simulink model "Model_DesktopSim"  (R2016b)
settings: Solver=ode3  StartTime=0.0  StopTime=180  FixedStep=Ts  MaxStep=Ts  RelTol=1e-4  EnableMultiTasking=on
InitFcn:
  | initSimScript();
values from neighbouring files (symbols this model uses):
  Ts = 80e-6*2    (= 0.00016)    [initSimScript.m]
undefined symbols (not defined in the file or in its folder): DiscIntNeverNeededParam
libraries: cables_lib x34, modbus_lib x21, simulink x18, transformer_lib x13, dynamic_load_lib x12, powerlib x6, discretizing x4, Batt_lib x1, PV_lib x1
(part 1 of 3)
settings Model: SimulationMode=accelerator  Creator=jlesage  LastModifiedBy=jlesage
settings SolverCC: EnableConcurrentExecution=on
settings DataIOCC: SaveFormat=StructureWithTime
settings OptimizationCC: BlockReduction=off  OptimizeBlockIOStorage=off  BufferReuse=off  GlobalBufferReuse=off  ExpressionFolding=off  LocalBlockOutputs=off
settings DebuggingCC: ParameterPrecisionLossMsg=none
settings HardwareCC: ProdBitPerPointer=32  ProdBitPerSizeT=32  ProdBitPerPtrDiffT=32  ProdLargestAtomicFloat=None  ProdWordSize=32  ProdLongLongMode=on  ProdHWDeviceType=Generic->32-bit x86 compatible
settings RTWCC: SystemTargetFile=slrt.tlc  TemplateMakefile=slrt_default_tmf  Description=Simulink Real-Time  RTWCompilerOptimization=on

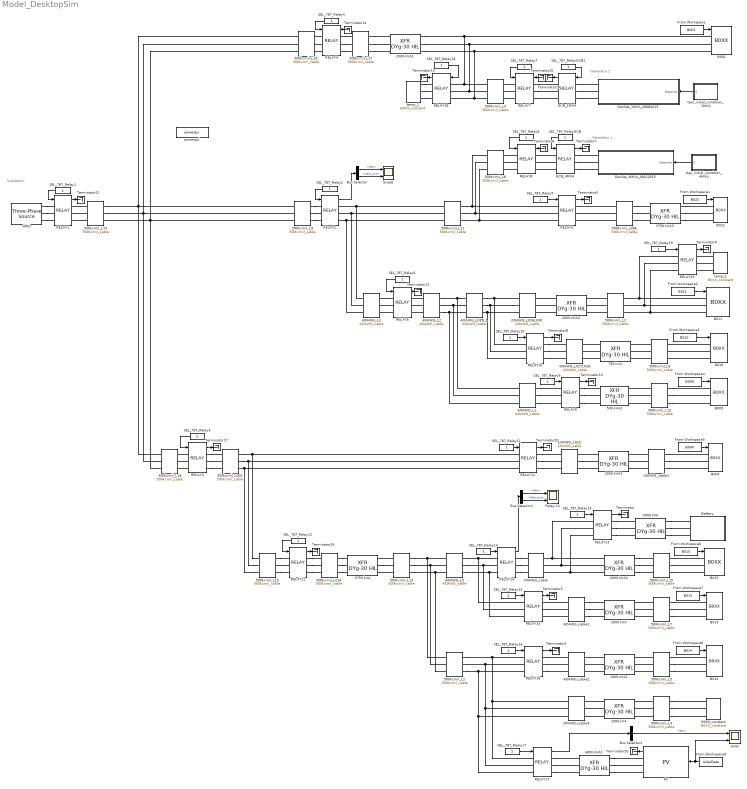
== system Model_DesktopSim ==
  note: Generator 2
  note: Generator 1
  note: Substation
  1/0AWG_L022 : cables_lib/1//0AWG_cable  length=1000  par_sets=1
  1/0AWG_cable1 : cables_lib/1//0AWG_cable  length=51  par_sets=1
  1000 kVA : transformer_lib/XFR DYg-30 HIL  Rating=1000  Vp=4160  Vs=460  Z=5.18  XR=2.5
  1000 kVA1 : transformer_lib/XFR DYg-30 HIL  Rating=1000  Vp=4160  Vs=216  Z=5.18  XR=2.5
  2/0AWG_L026L030 : cables_lib/2//0AWG_cable  length=1010  par_sets=1
  2000 kVA : transformer_lib/XFR DYg-30 HIL  Rating=2000  Vp=4160  Vs=216  Z=5.18  XR=2.5
  2000 kVA1 : transformer_lib/XFR DYg-30 HIL  Rating=2000  Vp=13800  Vs=460  Z=5.75  XR=5.7
  2000 kVA2 : transformer_lib/XFR DYg-30 HIL  Rating=2000  Vp=13800  Vs=460  Z=5.75  XR=5.7
  2000 kVA3 : transformer_lib/XFR DYg-30 HIL  Rating=2000  Vp=13800  Vs=460  Z=5.18  XR=2.5
  2000 kVA4 : transformer_lib/XFR DYg-30 HIL  Rating=2000  Vp=4160  Vs=216  Z=5.18  XR=2.5
  3750 kVA : transformer_lib/XFR DYg-30 HIL  Rating=3750  Vp=13800  Vs=4160  Z=4.75  XR=11.4
  3750 kVA3 : transformer_lib/XFR DYg-30 HIL  Rating=3750  Vp=13800  Vs=460  Z=4.75  XR=11.4
  4/0AWG_L027L028 : cables_lib/4//0AWG_cable  length=100  par_sets=1
  4/0AWG_L035L1 : cables_lib/4//0AWG_cable  length=1400  par_sets=1
  4/0AWG_L1 : cables_lib/4//0AWG_cable  length=25  par_sets=1
  4/0AWG_L2 : cables_lib/4//0AWG_cable  length=10  par_sets=1
  4/0AWG_L3 : cables_lib/4//0AWG_cable  length=150  par_sets=1
  4/0AWG_L5 : cables_lib/4//0AWG_cable  length=20  par_sets=1
  4/0AWG_cable{,1..3} (4 alike) : cables_lib/4//0AWG_cable  length=51  par_sets=1
  4000 kVA : transformer_lib/XFR DYg-30 HIL  Rating=4000  Vp=2047  Vs=4160  Z=6.37  XR=3.5
  4000 kVA1 : transformer_lib/XFR DYg-30 HIL  Rating=4000  Vp=2047  Vs=4160  Z=6.37  XR=3.5
  500 kVA2 : transformer_lib/XFR DYg-30 HIL  Rating=500  Vp=13800  Vs=460  Z=5  XR=4.9
  500kcmil_L002 : cables_lib/500kcmil_cable  length=1851  par_sets=1
  500kcmil_L006 : cables_lib/500kcmil_cable  length=251  par_sets=1
  500kcmil_L018 : cables_lib/500kcmil_cable  length=1851  par_sets=1
  500kcmil_L{1,6,15..16} (4 alike) : cables_lib/500kcmil_cable  length=50  par_sets=1
  500kcmil_L{4..5,7,10} (4 alike) : cables_lib/500kcmil_cable  length=25  par_sets=1
  500kcmil_L11 : cables_lib/500kcmil_cable  length=21  par_sets=1
  500kcmil_L12 : cables_lib/500kcmil_cable  length=50  par_sets=2
  500kcmil_L13 : cables_lib/500kcmil_cable  length=51  par_sets=1
  500kcmil_L14 : cables_lib/500kcmil_cable  length=350  par_sets=1
  500kcmil_L17 : cables_lib/500kcmil_cable  length=1000  par_sets=1
  500kcmil_L18 : cables_lib/500kcmil_cable  length=51  par_sets=1
  500kcmil_L2 : cables_lib/500kcmil_cable  length=125  par_sets=2
  500kcmil_L3 : cables_lib/500kcmil_cable  length=60  par_sets=1
  500kcmil_L8 : cables_lib/500kcmil_cable  length=100  par_sets=1
  500kcmil_L9 : cables_lib/500kcmil_cable  length=720  par_sets=1
  750 kVA : transformer_lib/XFR DYg-30 HIL  Rating=750  Vp=13800  Vs=460  Z=5.57  XR=3.96
  B001 : dynamic_load_lib/B0XX  V=460  P_Scale=2  Q_Scale=2
  B003_constant : dynamic_load_lib/B0XX_constant  v=460  kVA=60  pf=0.9
  B004 : dynamic_load_lib/B0XX  V=460  P_Scale=2  Q_Scale=2
  B009 : dynamic_load_lib/B0XX  V=460  P_Scale=2  Q_Scale=2
  B010 : dynamic_load_lib/B0XX  V=460  P_Scale=1  Q_Scale=1
  B011 : dynamic_load_lib/B0XX  V=460  P_Scale=1  Q_Scale=1
  B013 : dynamic_load_lib/B0XX  V=208  P_Scale=2  Q_Scale=2
  B014 : dynamic_load_lib/B0XX  V=208  P_Scale=1  Q_Scale=1
  B015 : dynamic_load_lib/B0XX  V=208  P_Scale=2  Q_Scale=2
  B022 : dynamic_load_lib/B0XX  V=460  P_Scale=1  Q_Scale=1
  Battery : Subsystem
  Bus Selector : BusSelector  OutputSignals=Iabc,Vabc_bus
  Bus Selector1 : BusSelector  OutputSignals=Iabc,Vabc_bus
  Bus Selector2 : BusSelector  OutputSignals=Iabc
  From Workspace : FromWorkspace  VariableName=B001  SampleTime=Ts  OutputAfterFinalValue=Holding final value
  From Workspace1 : FromWorkspace  VariableName=B022  SampleTime=Ts  OutputAfterFinalValue=Holding final value
  From Workspace2 : FromWorkspace  VariableName=B011  SampleTime=Ts  OutputAfterFinalValue=Holding final value
  From Workspace3 : FromWorkspace  VariableName=B010  SampleTime=Ts  OutputAfterFinalValue=Holding final value
  From Workspace4 : FromWorkspace  VariableName=B009  SampleTime=Ts  OutputAfterFinalValue=Holding final value
  From Workspace5 : FromWorkspace  VariableName=B004  SampleTime=Ts  OutputAfterFinalValue=Holding final value
  From Workspace6 : FromWorkspace  VariableName=B015  SampleTime=Ts  OutputAfterFinalValue=Holding final value
  From Workspace7 : FromWorkspace  VariableName=B013  SampleTime=Ts  OutputAfterFinalValue=Holding final value
  From Workspace8 : FromWorkspace  VariableName=B014  SampleTime=Ts  OutputAfterFinalValue=Holding final value
  From Workspace9 : FromWorkspace  VariableName=solarData  SampleTime=Ts  OutputAfterFinalValue=Holding final value
  GCB_1MVA : modbus_lib/RELAY  Ts=Ts
      link override Three-Phase V-I Measurement/Model/VI/Ia: GotoTag=LibraryTag_Ia
      link override Three-Phase V-I Measurement/Model/VI/Ib: GotoTag=LibraryTag_Ib
      link override Three-Phase V-I Measurement/Model/VI/Ic: GotoTag=LibraryTag_Ic
      link override Three-Phase V-I Measurement/Model/VI/Va: GotoTag=LibraryTag_Va
      link override Three-Phase V-I Measurement/Model/VI/Vb: GotoTag=LibraryTag_Vb
      link override Three-Phase V-I Measurement/Model/VI/Vc: GotoTag=LibraryTag_Vc
      link override Three-Phase V-I Measurement1/Model/VI/Ia: GotoTag=LibraryTag_Ia
      link override Three-Phase V-I Measurement1/Model/VI/Ib: GotoTag=LibraryTag_Ib
      link override Three-Phase V-I Measurement1/Model/VI/Ic: GotoTag=LibraryTag_Ic
      link override Three-Phase V-I Measurement1/Model/VI/Va: GotoTag=LibraryTag_Va
      link override Three-Phase V-I Measurement1/Model/VI/Vb: GotoTag=LibraryTag_Vb
      link override Three-Phase V-I Measurement1/Model/VI/Vc: GotoTag=LibraryTag_Vc
  GCB_4MVA : modbus_lib/RELAY  Ts=Ts
      link override Three-Phase V-I Measurement/Model/VI/Ia: GotoTag=LibraryTag_Ia
      link override Three-Phase V-I Measurement/Model/VI/Ib: GotoTag=LibraryTag_Ib
      link override Three-Phase V-I Measurement/Model/VI/Ic: GotoTag=LibraryTag_Ic
      link override Three-Phase V-I Measurement/Model/VI/Va: GotoTag=LibraryTag_Va
      link override Three-Phase V-I Measurement/Model/VI/Vb: GotoTag=LibraryTag_Vb
      link override Three-Phase V-I Measurement/Model/VI/Vc: GotoTag=LibraryTag_Vc
      link override Three-Phase V-I Measurement1/Model/VI/Ia: GotoTag=LibraryTag_Ia
      link override Three-Phase V-I Measurement1/Model/VI/Ib: GotoTag=LibraryTag_Ib
      link override Three-Phase V-I Measurement1/Model/VI/Ic: GotoTag=LibraryTag_Ic
      link override Three-Phase V-I Measurement1/Model/VI/Va: GotoTag=LibraryTag_Va
      link override Three-Phase V-I Measurement1/Model/VI/Vb: GotoTag=LibraryTag_Vb
      link override Three-Phase V-I Measurement1/Model/VI/Vc: GotoTag=LibraryTag_Vc
  GRID : powerlib/Electrical Sources/Three-Phase Source  InternalConnection=Yg  VoltagePhases=off  Voltage=13970  PhaseAngle=0  Voltage_phases=[25e3 25e3 25e3]/sqrt(3)  PhaseAngles_phases=[0 -120 +120]  Frequency=60  NonIdealSource=on  SpecifyImpedance=on  Resistance=0.8929  Inductance=16.58e-3  ShortCircuitLevel=375e6  BaseVoltage=13800  XRratio=7.9  BusType=swing  Pref=0  Qref=0  Prefabc=[10e3, 10e3, 10e3]  Qrefabc=[0, 0, 0]  Qmin=-inf  Qmax=inf
  GenSet_1MVA_09082015 : Subsystem
  GenSet_4MVA_09212015 : Subsystem
  Gen_initial_condition_1MVA : Subsystem
  Gen_initial_condition_4MVA : Subsystem
  PV : PV_lib/PV  max_power=4e6  VacRMS=1200  VacRMS_limit_pu=[1.15 0.85]
  RELAY1 : modbus_lib/RELAY  Ts=Ts
      link override Three-Phase V-I Measurement/Model/VI/Ia: GotoTag=LibraryTag_Ia
      link override Three-Phase V-I Measurement/Model/VI/Ib: GotoTag=LibraryTag_Ib
      link override Three-Phase V-I Measurement/Model/VI/Ic: GotoTag=LibraryTag_Ic
      link override Three-Phase V-I Measurement/Model/VI/Va: GotoTag=LibraryTag_Va
      link override Three-Phase V-I Measurement/Model/VI/Vb: GotoTag=LibraryTag_Vb
      link override Three-Phase V-I Measurement/Model/VI/Vc: GotoTag=LibraryTag_Vc
      link override Three-Phase V-I Measurement1/Model/VI/Ia: GotoTag=LibraryTag_Ia
      link override Three-Phase V-I Measurement1/Model/VI/Ib: GotoTag=LibraryTag_Ib
      link override Three-Phase V-I Measurement1/Model/VI/Ic: GotoTag=LibraryTag_Ic
      link override Three-Phase V-I Measurement1/Model/VI/Va: GotoTag=LibraryTag_Va
      link override Three-Phase V-I Measurement1/Model/VI/Vb: GotoTag=LibraryTag_Vb
      link override Three-Phase V-I Measurement1/Model/VI/Vc: GotoTag=LibraryTag_Vc
  RELAY10 : modbus_lib/RELAY  Ts=Ts
      link override Three-Phase V-I Measurement/Model/VI/Ia: GotoTag=LibraryTag_Ia
      link override Three-Phase V-I Measurement/Model/VI/Ib: GotoTag=LibraryTag_Ib
      link override Three-Phase V-I Measurement/Model/VI/Ic: GotoTag=LibraryTag_Ic
      link override Three-Phase V-I Measurement/Model/VI/Va: GotoTag=LibraryTag_Va
      link override Three-Phase V-I Measurement/Model/VI/Vb: GotoTag=LibraryTag_Vb
      link override Three-Phase V-I Measurement/Model/VI/Vc: GotoTag=LibraryTag_Vc
      link override Three-Phase V-I Measurement1/Model/VI/Ia: GotoTag=LibraryTag_Ia
      link override Three-Phase V-I Measurement1/Model/VI/Ib: GotoTag=LibraryTag_Ib
      link override Three-Phase V-I Measurement1/Model/VI/Ic: GotoTag=LibraryTag_Ic
      link override Three-Phase V-I Measurement1/Model/VI/Va: GotoTag=LibraryTag_Va
      link override Three-Phase V-I Measurement1/Model/VI/Vb: GotoTag=LibraryTag_Vb
      link override Three-Phase V-I Measurement1/Model/VI/Vc: GotoTag=LibraryTag_Vc
  RELAY11 : modbus_lib/RELAY  Ts=Ts
      link override Three-Phase V-I Measurement/Model/VI/Ia: GotoTag=LibraryTag_Ia
      link override Three-Phase V-I Measurement/Model/VI/Ib: GotoTag=LibraryTag_Ib
      link override Three-Phase V-I Measurement/Model/VI/Ic: GotoTag=LibraryTag_Ic
      link override Three-Phase V-I Measurement/Model/VI/Va: GotoTag=LibraryTag_Va
      link override Three-Phase V-I Measurement/Model/VI/Vb: GotoTag=LibraryTag_Vb
      link override Three-Phase V-I Measurement/Model/VI/Vc: GotoTag=LibraryTag_Vc
      link override Three-Phase V-I Measurement1/Model/VI/Ia: GotoTag=LibraryTag_Ia
      link override Three-Phase V-I Measurement1/Model/VI/Ib: GotoTag=LibraryTag_Ib
      link override Three-Phase V-I Measurement1/Model/VI/Ic: GotoTag=LibraryTag_Ic
      link override Three-Phase V-I Measurement1/Model/VI/Va: GotoTag=LibraryTag_Va
      link override Three-Phase V-I Measurement1/Model/VI/Vb: GotoTag=LibraryTag_Vb
      link override Three-Phase V-I Measurement1/Model/VI/Vc: GotoTag=LibraryTag_Vc
  RELAY12 : modbus_lib/RELAY  Ts=Ts
      link override Three-Phase V-I Measurement/Model/VI/Ia: GotoTag=LibraryTag_Ia
      link override Three-Phase V-I Measurement/Model/VI/Ib: GotoTag=LibraryTag_Ib
      link override Three-Phase V-I Measurement/Model/VI/Ic: GotoTag=LibraryTag_Ic
      link override Three-Phase V-I Measurement/Model/VI/Va: GotoTag=LibraryTag_Va
      link override Three-Phase V-I Measurement/Model/VI/Vb: GotoTag=LibraryTag_Vb
      link override Three-Phase V-I Measurement/Model/VI/Vc: GotoTag=LibraryTag_Vc
      link override Three-Phase V-I Measurement1/Model/VI/Ia: GotoTag=LibraryTag_Ia
      link override Three-Phase V-I Measurement1/Model/VI/Ib: GotoTag=LibraryTag_Ib
      link override Three-Phase V-I Measurement1/Model/VI/Ic: GotoTag=LibraryTag_Ic
      link override Three-Phase V-I Measurement1/Model/VI/Va: GotoTag=LibraryTag_Va
      link override Three-Phase V-I Measurement1/Model/VI/Vb: GotoTag=LibraryTag_Vb
      link override Three-Phase V-I Measurement1/Model/VI/Vc: GotoTag=LibraryTag_Vc
  RELAY13 : modbus_lib/RELAY  Ts=Ts
  RELAY14 : modbus_lib/RELAY  Ts=Ts
      link override Three-Phase V-I Measurement/Model/VI/Ia: GotoTag=LibraryTag_Ia
      link override Three-Phase V-I Measurement/Model/VI/Ib: GotoTag=LibraryTag_Ib
      link override Three-Phase V-I Measurement/Model/VI/Ic: GotoTag=LibraryTag_Ic
      link override Three-Phase V-I Measurement/Model/VI/Va: GotoTag=LibraryTag_Va
      link override Three-Phase V-I Measurement/Model/VI/Vb: GotoTag=LibraryTag_Vb
      link override Three-Phase V-I Measurement/Model/VI/Vc: GotoTag=LibraryTag_Vc
      link override Three-Phase V-I Measurement1/Model/VI/Ia: GotoTag=LibraryTag_Ia
      link override Three-Phase V-I Measurement1/Model/VI/Ib: GotoTag=LibraryTag_Ib
      link override Three-Phase V-I Measurement1/Model/VI/Ic: GotoTag=LibraryTag_Ic
      link override Three-Phase V-I Measurement1/Model/VI/Va: GotoTag=LibraryTag_Va
      link override Three-Phase V-I Measurement1/Model/VI/Vb: GotoTag=LibraryTag_Vb
      link override Three-Phase V-I Measurement1/Model/VI/Vc: GotoTag=LibraryTag_Vc
  RELAY15 : modbus_lib/RELAY  Ts=Ts
      link override Three-Phase V-I Measurement/Model/VI/Ia: GotoTag=LibraryTag_Ia
      link override Three-Phase V-I Measurement/Model/VI/Ib: GotoTag=LibraryTag_Ib
      link override Three-Phase V-I Measurement/Model/VI/Ic: GotoTag=LibraryTag_Ic
      link override Three-Phase V-I Measurement/Model/VI/Va: GotoTag=LibraryTag_Va
      link override Three-Phase V-I Measurement/Model/VI/Vb: GotoTag=LibraryTag_Vb
      link override Three-Phase V-I Measurement/Model/VI/Vc: GotoTag=LibraryTag_Vc
      link override Three-Phase V-I Measurement1/Model/VI/Ia: GotoTag=LibraryTag_Ia
      link override Three-Phase V-I Measurement1/Model/VI/Ib: GotoTag=LibraryTag_Ib
      link override Three-Phase V-I Measurement1/Model/VI/Ic: GotoTag=LibraryTag_Ic
      link override Three-Phase V-I Measurement1/Model/VI/Va: GotoTag=LibraryTag_Va
      link override Three-Phase V-I Measurement1/Model/VI/Vb: GotoTag=LibraryTag_Vb
      link override Three-Phase V-I Measurement1/Model/VI/Vc: GotoTag=LibraryTag_Vc
  RELAY16 : modbus_lib/RELAY  Ts=Ts
      link override Three-Phase V-I Measurement/Model/VI/Ia: GotoTag=LibraryTag_Ia
      link override Three-Phase V-I Measurement/Model/VI/Ib: GotoTag=LibraryTag_Ib
      link override Three-Phase V-I Measurement/Model/VI/Ic: GotoTag=LibraryTag_Ic
      link override Three-Phase V-I Measurement/Model/VI/Va: GotoTag=LibraryTag_Va
      link override Three-Phase V-I Measurement/Model/VI/Vb: GotoTag=LibraryTag_Vb
      link override Three-Phase V-I Measurement/Model/VI/Vc: GotoTag=LibraryTag_Vc
      link override Three-Phase V-I Measurement1/Model/VI/Ia: GotoTag=LibraryTag_Ia
      link override Three-Phase V-I Measurement1/Model/VI/Ib: GotoTag=LibraryTag_Ib
      link override Three-Phase V-I Measurement1/Model/VI/Ic: GotoTag=LibraryTag_Ic
      link override Three-Phase V-I Measurement1/Model/VI/Va: GotoTag=LibraryTag_Va
      link override Three-Phase V-I Measurement1/Model/VI/Vb: GotoTag=LibraryTag_Vb
      link override Three-Phase V-I Measurement1/Model/VI/Vc: GotoTag=LibraryTag_Vc
  RELAY17 : modbus_lib/RELAY  Ts=Ts
      link override Three-Phase V-I Measurement/Model/VI/Ia: GotoTag=LibraryTag_Ia
      link override Three-Phase V-I Measurement/Model/VI/Ib: GotoTag=LibraryTag_Ib
      link override Three-Phase V-I Measurement/Model/VI/Ic: GotoTag=LibraryTag_Ic
      link override Three-Phase V-I Measurement/Model/VI/Va: GotoTag=LibraryTag_Va
      link override Three-Phase V-I Measurement/Model/VI/Vb: GotoTag=LibraryTag_Vb
      link override Three-Phase V-I Measurement/Model/VI/Vc: GotoTag=LibraryTag_Vc
      link override Three-Phase V-I Measurement1/Model/VI/Ia: GotoTag=LibraryTag_Ia
      link override Three-Phase V-I Measurement1/Model/VI/Ib: GotoTag=LibraryTag_Ib
      link override Three-Phase V-I Measurement1/Model/VI/Ic: GotoTag=LibraryTag_Ic
      link override Three-Phase V-I Measurement1/Model/VI/Va: GotoTag=LibraryTag_Va
      link override Three-Phase V-I Measurement1/Model/VI/Vb: GotoTag=LibraryTag_Vb
      link override Three-Phase V-I Measurement1/Model/VI/Vc: GotoTag=LibraryTag_Vc
  RELAY18 : modbus_lib/RELAY  Ts=Ts
      link override Three-Phase V-I Measurement/Model/VI/Ia: GotoTag=LibraryTag_Ia
      link override Three-Phase V-I Measurement/Model/VI/Ib: GotoTag=LibraryTag_Ib
      link override Three-Phase V-I Measurement/Model/VI/Ic: GotoTag=LibraryTag_Ic
      link override Three-Phase V-I Measurement/Model/VI/Va: GotoTag=LibraryTag_Va
      link override Three-Phase V-I Measurement/Model/VI/Vb: GotoTag=LibraryTag_Vb
      link override Three-Phase V-I Measurement/Model/VI/Vc: GotoTag=LibraryTag_Vc
      link override Three-Phase V-I Measurement1/Model/VI/Ia: GotoTag=LibraryTag_Ia
      link override Three-Phase V-I Measurement1/Model/VI/Ib: GotoTag=LibraryTag_Ib
      link override Three-Phase V-I Measurement1/Model/VI/Ic: GotoTag=LibraryTag_Ic
      link override Three-Phase V-I Measurement1/Model/VI/Va: GotoTag=LibraryTag_Va
      link override Three-Phase V-I Measurement1/Model/VI/Vb: GotoTag=LibraryTag_Vb
      link override Three-Phase V-I Measurement1/Model/VI/Vc: GotoTag=LibraryTag_Vc
  RELAY19 : modbus_lib/RELAY  Ts=Ts
      link override Three-Phase V-I Measurement/Model/VI/Ia: GotoTag=LibraryTag_Ia
      link override Three-Phase V-I Measurement/Model/VI/Ib: GotoTag=LibraryTag_Ib
      link override Three-Phase V-I Measurement/Model/VI/Ic: GotoTag=LibraryTag_Ic
      link override Three-Phase V-I Measurement/Model/VI/Va: GotoTag=LibraryTag_Va
      link override Three-Phase V-I Measurement/Model/VI/Vb: GotoTag=LibraryTag_Vb
      link override Three-Phase V-I Measurement/Model/VI/Vc: GotoTag=LibraryTag_Vc
      link override Three-Phase V-I Measurement1/Model/VI/Ia: GotoTag=LibraryTag_Ia
      link override Three-Phase V-I Measurement1/Model/VI/Ib: GotoTag=LibraryTag_Ib
      link override Three-Phase V-I Measurement1/Model/VI/Ic: GotoTag=LibraryTag_Ic
      link override Three-Phase V-I Measurement1/Model/VI/Va: GotoTag=LibraryTag_Va
      link override Three-Phase V-I Measurement1/Model/VI/Vb: GotoTag=LibraryTag_Vb
      link override Three-Phase V-I Measurement1/Model/VI/Vc: GotoTag=LibraryTag_Vc
  RELAY2 : modbus_lib/RELAY  Ts=Ts
      link override Three-Phase V-I Measurement/Model/VI/Ia: GotoTag=LibraryTag_Ia
      link override Three-Phase V-I Measurement/Model/VI/Ib: GotoTag=LibraryTag_Ib
      link override Three-Phase V-I Measurement/Model/VI/Ic: GotoTag=LibraryTag_Ic
      link override Three-Phase V-I Measurement/Model/VI/Va: GotoTag=LibraryTag_Va
      link override Three-Phase V-I Measurement/Model/VI/Vb: GotoTag=LibraryTag_Vb
      link override Three-Phase V-I Measurement/Model/VI/Vc: GotoTag=LibraryTag_Vc
      link override Three-Phase V-I Measurement1/Model/VI/Ia: GotoTag=LibraryTag_Ia
      link override Three-Phase V-I Measurement1/Model/VI/Ib: GotoTag=LibraryTag_Ib
      link override Three-Phase V-I Measurement1/Model/VI/Ic: GotoTag=LibraryTag_Ic
      link override Three-Phase V-I Measurement1/Model/VI/Va: GotoTag=LibraryTag_Va
      link override Three-Phase V-I Measurement1/Model/VI/Vb: GotoTag=LibraryTag_Vb
      link override Three-Phase V-I Measurement1/Model/VI/Vc: GotoTag=LibraryTag_Vc
  RELAY3 : modbus_lib/RELAY  Ts=Ts
      link override Three-Phase V-I Measurement/Model/VI/Ia: GotoTag=LibraryTag_Ia
      link override Three-Phase V-I Measurement/Model/VI/Ib: GotoTag=LibraryTag_Ib
      link override Three-Phase V-I Measurement/Model/VI/Ic: GotoTag=LibraryTag_Ic
      link override Three-Phase V-I Measurement/Model/VI/Va: GotoTag=LibraryTag_Va
      link override Three-Phase V-I Measurement/Model/VI/Vb: GotoTag=LibraryTag_Vb
      link override Three-Phase V-I Measurement/Model/VI/Vc: GotoTag=LibraryTag_Vc
      link override Three-Phase V-I Measurement1/Model/VI/Ia: GotoTag=LibraryTag_Ia
      link override Three-Phase V-I Measurement1/Model/VI/Ib: GotoTag=LibraryTag_Ib
      link override Three-Phase V-I Measurement1/Model/VI/Ic: GotoTag=LibraryTag_Ic
      link override Three-Phase V-I Measurement1/Model/VI/Va: GotoTag=LibraryTag_Va
      link override Three-Phase V-I Measurement1/Model/VI/Vb: GotoTag=LibraryTag_Vb
      link override Three-Phase V-I Measurement1/Model/VI/Vc: GotoTag=LibraryTag_Vc
  RELAY4 : modbus_lib/RELAY  Ts=Ts
      link override Three-Phase V-I Measurement/Model/VI/Ia: GotoTag=LibraryTag_Ia
      link override Three-Phase V-I Measurement/Model/VI/Ib: GotoTag=LibraryTag_Ib
      link override Three-Phase V-I Measurement/Model/VI/Ic: GotoTag=LibraryTag_Ic
      link override Three-Phase V-I Measurement/Model/VI/Va: GotoTag=LibraryTag_Va
      link override Three-Phase V-I Measurement/Model/VI/Vb: GotoTag=LibraryTag_Vb
      link override Three-Phase V-I Measurement/Model/VI/Vc: GotoTag=LibraryTag_Vc
      link override Three-Phase V-I Measurement1/Model/VI/Ia: GotoTag=LibraryTag_Ia
      link override Three-Phase V-I Measurement1/Model/VI/Ib: GotoTag=LibraryTag_Ib
      link override Three-Phase V-I Measurement1/Model/VI/Ic: GotoTag=LibraryTag_Ic
      link override Three-Phase V-I Measurement1/Model/VI/Va: GotoTag=LibraryTag_Va
      link override Three-Phase V-I Measurement1/Model/VI/Vb: GotoTag=LibraryTag_Vb
      link override Three-Phase V-I Measurement1/Model/VI/Vc: GotoTag=LibraryTag_Vc
  RELAY5 : modbus_lib/RELAY  Ts=Ts
      link override Three-Phase V-I Measurement/Model/VI/Ia: GotoTag=LibraryTag_Ia
      link override Three-Phase V-I Measurement/Model/VI/Ib: GotoTag=LibraryTag_Ib
      link override Three-Phase V-I Measurement/Model/VI/Ic: GotoTag=LibraryTag_Ic
      link override Three-Phase V-I Measurement/Model/VI/Va: GotoTag=LibraryTag_Va
      link override Three-Phase V-I Measurement/Model/VI/Vb: GotoTag=LibraryTag_Vb
      link override Three-Phase V-I Measurement/Model/VI/Vc: GotoTag=LibraryTag_Vc
      link override Three-Phase V-I Measurement1/Model/VI/Ia: GotoTag=LibraryTag_Ia
      link override Three-Phase V-I Measurement1/Model/VI/Ib: GotoTag=LibraryTag_Ib
      link override Three-Phase V-I Measurement1/Model/VI/Ic: GotoTag=LibraryTag_Ic
      link override Three-Phase V-I Measurement1/Model/VI/Va: GotoTag=LibraryTag_Va
      link override Three-Phase V-I Measurement1/Model/VI/Vb: GotoTag=LibraryTag_Vb
      link override Three-Phase V-I Measurement1/Model/VI/Vc: GotoTag=LibraryTag_Vc
  RELAY6 : modbus_lib/RELAY  Ts=Ts
      link override Three-Phase V-I Measurement/Model/VI/Ia: GotoTag=LibraryTag_Ia
      link override Three-Phase V-I Measurement/Model/VI/Ib: GotoTag=LibraryTag_Ib
      link override Three-Phase V-I Measurement/Model/VI/Ic: GotoTag=LibraryTag_Ic
      link override Three-Phase V-I Measurement/Model/VI/Va: GotoTag=LibraryTag_Va
      link override Three-Phase V-I Measurement/Model/VI/Vb: GotoTag=LibraryTag_Vb
      link override Three-Phase V-I Measurement/Model/VI/Vc: GotoTag=LibraryTag_Vc
      link override Three-Phase V-I Measurement1/Model/VI/Ia: GotoTag=LibraryTag_Ia
      link override Three-Phase V-I Measurement1/Model/VI/Ib: GotoTag=LibraryTag_Ib
      link override Three-Phase V-I Measurement1/Model/VI/Ic: GotoTag=LibraryTag_Ic
      link override Three-Phase V-I Measurement1/Model/VI/Va: GotoTag=LibraryTag_Va
      link override Three-Phase V-I Measurement1/Model/VI/Vb: GotoTag=LibraryTag_Vb
      link override Three-Phase V-I Measurement1/Model/VI/Vc: GotoTag=LibraryTag_Vc
  RELAY7 : modbus_lib/RELAY  Ts=Ts
      link override Three-Phase V-I Measurement/Model/VI/Ia: GotoTag=LibraryTag_Ia
      link override Three-Phase V-I Measurement/Model/VI/Ib: GotoTag=LibraryTag_Ib
      link override Three-Phase V-I Measurement/Model/VI/Ic: GotoTag=LibraryTag_Ic
      link override Three-Phase V-I Measurement/Model/VI/Va: GotoTag=LibraryTag_Va
      link override Three-Phase V-I Measurement/Model/VI/Vb: GotoTag=LibraryTag_Vb
      link override Three-Phase V-I Measurement/Model/VI/Vc: GotoTag=LibraryTag_Vc
      link override Three-Phase V-I Measurement1/Model/VI/Ia: GotoTag=LibraryTag_Ia
      link override Three-Phase V-I Measurement1/Model/VI/Ib: GotoTag=LibraryTag_Ib
      link override Three-Phase V-I Measurement1/Model/VI/Ic: GotoTag=LibraryTag_Ic
      link override Three-Phase V-I Measurement1/Model/VI/Va: GotoTag=LibraryTag_Va
      link override Three-Phase V-I Measurement1/Model/VI/Vb: GotoTag=LibraryTag_Vb
      link override Three-Phase V-I Measurement1/Model/VI/Vc: GotoTag=LibraryTag_Vc
  RELAY8 : modbus_lib/RELAY  Ts=Ts
      link override Three-Phase V-I Measurement/Model/VI/Ia: GotoTag=LibraryTag_Ia
      link override Three-Phase V-I Measurement/Model/VI/Ib: GotoTag=LibraryTag_Ib
      link override Three-Phase V-I Measurement/Model/VI/Ic: GotoTag=LibraryTag_Ic
      link override Three-Phase V-I Measurement/Model/VI/Va: GotoTag=LibraryTag_Va
      link override Three-Phase V-I Measurement/Model/VI/Vb: GotoTag=LibraryTag_Vb
      link override Three-Phase V-I Measurement/Model/VI/Vc: GotoTag=LibraryTag_Vc
      link override Three-Phase V-I Measurement1/Model/VI/Ia: GotoTag=LibraryTag_Ia
      link override Three-Phase V-I Measurement1/Model/VI/Ib: GotoTag=LibraryTag_Ib
      link override Three-Phase V-I Measurement1/Model/VI/Ic: GotoTag=LibraryTag_Ic
      link override Three-Phase V-I Measurement1/Model/VI/Va: GotoTag=LibraryTag_Va
      link override Three-Phase V-I Measurement1/Model/VI/Vb: GotoTag=LibraryTag_Vb
      link override Three-Phase V-I Measurement1/Model/VI/Vc: GotoTag=LibraryTag_Vc
  RELAY9 : modbus_lib/RELAY  Ts=Ts
      link override Three-Phase V-I Measurement/Model/VI/Ia: GotoTag=LibraryTag_Ia
      link override Three-Phase V-I Measurement/Model/VI/Ib: GotoTag=LibraryTag_Ib
      link override Three-Phase V-I Measurement/Model/VI/Ic: GotoTag=LibraryTag_Ic
      link override Three-Phase V-I Measurement/Model/VI/Va: GotoTag=LibraryTag_Va
      link override Three-Phase V-I Measurement/Model/VI/Vb: GotoTag=LibraryTag_Vb
      link override Three-Phase V-I Measurement/Model/VI/Vc: GotoTag=LibraryTag_Vc
      link override Three-Phase V-I Measurement1/Model/VI/Ia: GotoTag=LibraryTag_Ia
      link override Three-Phase V-I Measurement1/Model/VI/Ib: GotoTag=LibraryTag_Ib
      link override Three-Phase V-I Measurement1/Model/VI/Ic: GotoTag=LibraryTag_Ic
      link override Three-Phase V-I Measurement1/Model/VI/Va: GotoTag=LibraryTag_Va
      link override Three-Phase V-I Measurement1/Model/VI/Vb: GotoTag=LibraryTag_Vb
      link override Three-Phase V-I Measurement1/Model/VI/Vc: GotoTag=LibraryTag_Vc
  Relay 14 : Scope  NumInputPorts=2
  SEL_787_Relay{1..19} (19 alike) : Constant
  SEL_787_RelayGCB : Constant
  SEL_787_RelayGCB1 : Constant
  Scope : Scope  NumInputPorts=2
  Solar : Scope  NumInputPorts=2
  Terminator{,2..3,5..11,13..21} (19 alike) : Terminator
  powergui : powerlib/powergui  Priority=2  SimulationMode=Discrete  SolverType=Tustin/Backward Euler (TBE)  SampleTime=Ts  frequency=60  SPID=off  DisableSnubberDevices=off  DisableRonSwitches=off  DisableVfSwitches=off  SwTol=0  DisplayEquations=off  Interpol=off  ExternalGateDelay=off  methode=off  Ts=0  FunctionMessages=off  echomessages=off  HookPort=off  EnableUseOfTLC=on  x0status=blocks  frequencyindice=0  Pbase=100e6  ErrMax=1e-4  Iterations=50  UnitsV=kV  UnitsW=MW  buscounter=0  RestoreLinks=warning  ResistiveCurrentMeasurement=off  Frange=logspace(0,3,50)  Ylog=off  Xlog=off  ShowGrid=off  save=off  variable=ZData  structure=0  ZoomFFT=on  StartTime=0.0  cycles=2  DisplayStyle=off  fundamental=60  FreqAxis=off  MaxFrequency=1000  frequencyindicesteady=1  RmsSteady=1  display=off
  temp_1 : dynamic_load_lib/B0XX_constant  v=460  kVA=100  pf=0.90
  temp_2 : dynamic_load_lib/B0XX_constant  v=460  kVA=100  pf=0.90
  wires:
  From Workspace9/1 -> Solar/2, PV/1
  From Workspace7/1 -> B013/1
  SEL_787_Relay15/1 -> RELAY15/1
  SEL_787_Relay14/1 -> RELAY14/1
  RELAY15/1 -> Terminator2/1
  SEL_787_Relay13/1 -> RELAY13/1
  From Workspace6/1 -> B015/1
  RELAY13/1 -> Terminator/1
  From Workspace8/1 -> B014/1
  RELAY16/1 -> Terminator3/1
  SEL_787_Relay16/1 -> RELAY16/1
  RELAY17/1 -> Bus Selector2/1
  SEL_787_Relay17/1 -> RELAY17/1
  Gen_initial_condition_1MVA/1(S) -> GenSet_1MVA_09082015/1(Setpoints)
  RELAY5/1 -> Terminator5/1
  SEL_787_Relay5/1 -> RELAY5/1
  SEL_787_Relay8/1 -> RELAY8/1
  SEL_787_RelayGCB/1 -> GCB_4MVA/1
  RELAY8/1 -> Terminator6/1
  GCB_4MVA/1 -> Terminator7/1
  Gen_initial_condition_4MVA/1(S) -> GenSet_4MVA_09212015/1(Setpoints)
  From Workspace1/1 -> B022/1
  RELAY10/1 -> Terminator8/1
  SEL_787_Relay10/1 -> RELAY10/1
  From Workspace3/1 -> B010/1
  From Workspace2/1 -> B011/1
  SEL_787_Relay19/1 -> RELAY19/1
  RELAY19/1 -> Terminator9/1
  SEL_787_Relay9/1 -> RELAY9/1
  RELAY9/1 -> Terminator10/1
  From Workspace4/1 -> B009/1
  RELAY6/1 -> Terminator11/1
  SEL_787_Relay6/1 -> RELAY6/1
  RELAY2/1 -> Bus Selector/1
  SEL_787_Relay2/1 -> RELAY2/1
  RELAY4/1 -> Terminator14/1
  SEL_787_Relay4/1 -> RELAY4/1
  RELAY7/1 -> Terminator15/1
  SEL_787_Relay7/1 -> RELAY7/1
  GCB_1MVA/1 -> Terminator16/1
  SEL_787_RelayGCB1/1 -> GCB_1MVA/1
  SEL_787_Relay18/1 -> RELAY18/1
  RELAY18/1 -> Terminator13/1
  RELAY3/1 -> Terminator17/1
  SEL_787_Relay3/1 -> RELAY3/1
  RELAY11/1 -> Terminator18/1
  SEL_787_Relay11/1 -> RELAY11/1
  From Workspace5/1 -> B004/1
  RELAY12/1 -> Terminator19/1
  SEL_787_Relay12/1 -> RELAY12/1
  PV/1 -> Terminator20/1
  RELAY1/1 -> Terminator21/1
  SEL_787_Relay1/1 -> RELAY1/1
  Bus Selector/1 -> Scope/1  "<Iabc>"
  Bus Selector/2 -> Scope/2  "<Vabc_bus>"
  RELAY14/1 -> Bus Selector1/1
  Bus Selector1/1 -> Relay 14/1  "<Iabc>"
  Bus Selector1/2 -> Relay 14/2  "<Vabc_bus>"
  From Workspace/1 -> B001/1
  Bus Selector2/1 -> Solar/1  "<Iabc>"
  connections:
  RELAY14/LConn3 -- 4/0AWG_L5/RConn3 -- RELAY15/LConn3
  RELAY14/LConn2 -- 4/0AWG_L5/RConn2 -- RELAY15/LConn2
  RELAY14/LConn1 -- 4/0AWG_L5/RConn1 -- RELAY15/LConn1
  4/0AWG_cable3/LConn3 -- RELAY17/LConn3 -- RELAY16/LConn3 -- 500kcmil_L1/RConn3
  4/0AWG_cable3/LConn1 -- RELAY17/LConn1 -- 500kcmil_L1/RConn1 -- RELAY16/LConn1
  4/0AWG_cable/RConn3 -- 2000 kVA4/LConn3 -- RELAY13/LConn3
  4/0AWG_cable/RConn2 -- 2000 kVA4/LConn2 -- RELAY13/LConn2
  4/0AWG_cable/RConn1 -- 2000 kVA4/LConn1 -- RELAY13/LConn1
  4/0AWG_cable3/LConn2 -- RELAY17/LConn2 -- RELAY16/LConn2 -- 500kcmil_L1/RConn2
  500kcmil_L13/RConn3 -- 500kcmil_L1/LConn3 -- 4/0AWG_L5/LConn3
  500kcmil_L13/RConn2 -- 500kcmil_L1/LConn2 -- 4/0AWG_L5/LConn2
  500kcmil_L13/RConn1 -- 500kcmil_L1/LConn1 -- 4/0AWG_L5/LConn1
  RELAY14/RConn3 -- 4/0AWG_cable/LConn3
  RELAY14/RConn1 -- 4/0AWG_cable/LConn1
  4000 kVA1/LConn3 -- PV/RConn3
  4000 kVA1/LConn2 -- PV/RConn2
  4000 kVA1/LConn1 -- PV/RConn1
  RELAY14/RConn2 -- 4/0AWG_cable/LConn2
  500kcmil_L10/RConn1 -- B015/LConn1
  500kcmil_L7/RConn2 -- B013/LConn2
  500kcmil_L10/RConn2 -- B015/LConn2
  500kcmil_L7/RConn1 -- B013/LConn1
  500kcmil_L10/RConn3 -- B015/LConn3
  RELAY15/RConn2 -- 4/0AWG_cable1/LConn2
  500kcmil_L4/RConn1 -- B003_constant/LConn1
  2000 kVA4/RConn3 -- 500kcmil_L10/LConn3
  4/0AWG_cable1/RConn1 -- 2000 kVA/LConn1
  500kcmil_L4/RConn3 -- B003_constant/LConn3
  4/0AWG_cable1/RConn2 -- 2000 kVA/LConn2
  RELAY16/RConn3 -- 4/0AWG_cable2/LConn3
  500kcmil_L5/LConn2 -- 1000 kVA1/RConn2
  RELAY16/RConn1 -- 4/0AWG_cable2/LConn1
  500kcmil_L4/LConn3 -- 1000 kVA/RConn3
  500kcmil_L4/RConn2 -- B003_constant/LConn2
  1000 kVA1/LConn3 -- 4/0AWG_cable2/RConn3
  4/0AWG_cable1/LConn3 -- RELAY15/RConn3
  4/0AWG_cable2/LConn2 -- RELAY16/RConn2
  500kcmil_L5/LConn1 -- 1000 kVA1/RConn1
  500kcmil_L7/LConn2 -- 2000 kVA/RConn2
  500kcmil_L5/LConn3 -- 1000 kVA1/RConn3
  1000 kVA1/LConn1 -- 4/0AWG_cable2/RConn1
  500kcmil_L7/LConn3 -- 2000 kVA/RConn3
  4/0AWG_cable1/LConn1 -- RELAY15/RConn1
  4/0AWG_cable1/RConn3 -- 2000 kVA/LConn3
  500kcmil_L7/LConn1 -- 2000 kVA/RConn1
  1000 kVA1/LConn2 -- 4/0AWG_cable2/RConn2
  2000 kVA4/RConn2 -- 500kcmil_L10/LConn2
  500kcmil_L4/LConn2 -- 1000 kVA/RConn2
  2000 kVA4/RConn1 -- 500kcmil_L10/LConn1
  500kcmil_L5/RConn1 -- B014/LConn1
  500kcmil_L5/RConn2 -- B014/LConn2
  500kcmil_L7/RConn3 -- B013/LConn3
  RELAY13/RConn3 -- 4000 kVA/RConn3
  500kcmil_L4/LConn1 -- 1000 kVA/RConn1
  1000 kVA/LConn2 -- 4/0AWG_cable3/RConn2
  RELAY17/RConn2 -- 4000 kVA1/RConn2
  RELAY17/RConn1 -- 4000 kVA1/RConn1
  1000 kVA/LConn3 -- 4/0AWG_cable3/RConn3
  RELAY17/RConn3 -- 4000 kVA1/RConn3
  1000 kVA/LConn1 -- 4/0AWG_cable3/RConn1
  500kcmil_L5/RConn3 -- B014/LConn3
  RELAY13/RConn2 -- 4000 kVA/RConn2
  RELAY13/RConn1 -- 4000 kVA/RConn1
  2/0AWG_L026L030/LConn2 -- 4/0AWG_L035L1/RConn2 -- RELAY10/LConn2
  2/0AWG_L026L030/LConn3 -- 4/0AWG_L035L1/RConn3 -- RELAY10/LConn3
  2/0AWG_L026L030/LConn1 -- RELAY10/LConn1 -- 4/0AWG_L035L1/RConn1
  500kcmil_L11/RConn3 -- 500kcmil_L8/RConn3 -- RELAY5/LConn3
  500kcmil_L11/RConn2 -- 500kcmil_L8/RConn2 -- RELAY5/LConn2
  500kcmil_L11/RConn1 -- 500kcmil_L8/RConn1 -- RELAY5/LConn1
  4/0AWG_L035L1/LConn2 -- 4/0AWG_L2/RConn2 -- 4/0AWG_L1/LConn2
  RELAY19/LConn3 -- B011/LConn3 -- 500kcmil_L2/RConn3
  RELAY19/LConn2 -- B011/LConn2 -- 500kcmil_L2/RConn2
  RELAY19/LConn1 -- B011/LConn1 -- 500kcmil_L2/RConn1
  4/0AWG_L035L1/LConn3 -- 4/0AWG_L2/RConn3 -- 4/0AWG_L1/LConn3
  4/0AWG_L035L1/LConn1 -- 4/0AWG_L2/RConn1 -- 4/0AWG_L1/LConn1
  500kcmil_L006/LConn3 -- RELAY5/RConn3
  500kcmil_L006/LConn2 -- RELAY5/RConn2
  500kcmil_L006/LConn1 -- RELAY5/RConn1
  RELAY6/LConn1 -- 4/0AWG_L3/RConn1
  RELAY6/LConn2 -- 4/0AWG_L3/RConn2
  RELAY6/LConn3 -- 4/0AWG_L3/RConn3
  500kcmil_L12/LConn3 -- 500 kVA2/RConn3
  500kcmil_L12/LConn2 -- 500 kVA2/RConn2
  500kcmil_L12/LConn1 -- 500 kVA2/RConn1
  750 kVA/LConn1 -- 4/0AWG_L027L028/RConn1
  750 kVA/LConn2 -- 4/0AWG_L027L028/RConn2
  750 kVA/LConn3 -- 4/0AWG_L027L028/RConn3
  2000 kVA2/LConn1 -- 2/0AWG_L026L030/RConn1
  2000 kVA2/LConn2 -- 2/0AWG_L026L030/RConn2
  2000 kVA2/LConn3 -- 2/0AWG_L026L030/RConn3
  B010/LConn1 -- 500kcmil_L6/RConn1
  B010/LConn2 -- 500kcmil_L6/RConn2
  B010/LConn3 -- 500kcmil_L6/RConn3
  500kcmil_L6/LConn1 -- 750 kVA/RConn1
  500kcmil_L6/LConn2 -- 750 kVA/RConn2
  500kcmil_L6/LConn3 -- 750 kVA/RConn3
  500kcmil_L2/LConn3 -- 2000 kVA2/RConn3
  500kcmil_L2/LConn2 -- 2000 kVA2/RConn2
  500kcmil_L2/LConn1 -- 2000 kVA2/RConn1
  3750 kVA3/RConn3 -- B022/LConn3
  3750 kVA3/RConn2 -- B022/LConn2
  3750 kVA3/RConn1 -- B022/LConn1
  RELAY10/RConn3 -- 4/0AWG_L027L028/LConn3
  RELAY10/RConn2 -- 4/0AWG_L027L028/LConn2
  RELAY10/RConn1 -- 4/0AWG_L027L028/LConn1
  RELAY9/RConn3 -- 500 kVA2/LConn3
  RELAY9/RConn2 -- 500 kVA2/LConn2
  RELAY9/RConn1 -- 500 kVA2/LConn1
  4/0AWG_L1/RConn3 -- RELAY9/LConn3
  4/0AWG_L1/RConn2 -- RELAY9/LConn2
  4/0AWG_L1/RConn1 -- RELAY9/LConn1
  500kcmil_L12/RConn3 -- B009/LConn3
  500kcmil_L12/RConn2 -- B009/LConn2
  500kcmil_L12/RConn1 -- B009/LConn1
  500kcmil_L006/RConn3 -- 3750 kVA3/LConn3
  500kcmil_L006/RConn2 -- 3750 kVA3/LConn2
  500kcmil_L006/RConn1 -- 3750 kVA3/LConn1
  4/0AWG_L2/LConn3 -- RELAY6/RConn3
  4/0AWG_L2/LConn2 -- RELAY6/RConn2
  4/0AWG_L2/LConn1 -- RELAY6/RConn1
  4/0AWG_L3/LConn2 -- 500kcmil_L11/LConn2 -- RELAY2/RConn2
  4/0AWG_L3/LConn3 -- 500kcmil_L11/LConn3 -- RELAY2/RConn3
  4/0AWG_L3/LConn1 -- 500kcmil_L11/LConn1 -- RELAY2/RConn1
  500kcmil_L9/RConn3 -- RELAY2/LConn3
  500kcmil_L9/RConn2 -- RELAY2/LConn2
  500kcmil_L9/RConn1 -- RELAY2/LConn1
  temp_1/LConn3 -- RELAY19/RConn3
  temp_1/LConn2 -- RELAY19/RConn2
  temp_1/LConn1 -- RELAY19/RConn1
  GRID/RConn3 -- RELAY1/LConn3
  GRID/RConn2 -- RELAY1/LConn2
  GRID/RConn1 -- RELAY1/LConn1
  500kcmil_L14/LConn3 -- RELAY1/RConn3
  500kcmil_L14/LConn2 -- RELAY1/RConn2
  500kcmil_L14/LConn1 -- RELAY1/RConn1
  500kcmil_L14/RConn1 -- 500kcmil_L18/LConn1 -- 500kcmil_L16/LConn1 -- 500kcmil_L9/LConn1
  500kcmil_L14/RConn2 -- 500kcmil_L18/LConn2 -- 500kcmil_L16/LConn2 -- 500kcmil_L9/LConn2
  500kcmil_L9/LConn3 -- 500kcmil_L18/LConn3 -- 500kcmil_L14/RConn3 -- 500kcmil_L16/LConn3
  RELAY8/LConn1 -- 500kcmil_L8/LConn1
  RELAY8/LConn2 -- 500kcmil_L8/LConn2
  RELAY8/LConn3 -- 500kcmil_L8/LConn3
  GCB_4MVA/LConn1 -- RELAY8/RConn1
  GCB_4MVA/LConn2 -- RELAY8/RConn2
  GCB_4MVA/LConn3 -- RELAY8/RConn3
  GCB_4MVA/RConn1 -- GenSet_4MVA_09212015/RConn1
  GCB_4MVA/RConn2 -- GenSet_4MVA_09212015/RConn2
  GCB_4MVA/RConn3 -- GenSet_4MVA_09212015/RConn3
  2000 kVA1/RConn1 -- B001/LConn1 -- 500kcmil_L3/RConn1 -- RELAY18/LConn1
  2000 kVA1/RConn2 -- B001/LConn2 -- 500kcmil_L3/RConn2 -- RELAY18/LConn2
  2000 kVA1/RConn3 -- B001/LConn3 -- 500kcmil_L3/RConn3 -- RELAY18/LConn3
  RELAY4/RConn2 -- 500kcmil_L17/LConn2
  RELAY4/RConn1 -- 500kcmil_L17/LConn1
  500kcmil_L17/RConn3 -- 2000 kVA1/LConn3
  RELAY4/RConn3 -- 500kcmil_L17/LConn3
  500kcmil_L17/RConn2 -- 2000 kVA1/LConn2
  500kcmil_L17/RConn1 -- 2000 kVA1/LConn1
  RELAY4/LConn2 -- 500kcmil_L16/RConn2
  RELAY4/LConn3 -- 500kcmil_L16/RConn3
  RELAY4/LConn1 -- 500kcmil_L16/RConn1
  RELAY7/LConn1 -- 500kcmil_L3/LConn1
  RELAY7/LConn2 -- 500kcmil_L3/LConn2
  RELAY7/LConn3 -- 500kcmil_L3/LConn3
  RELAY7/RConn1 -- GCB_1MVA/RConn1
  RELAY7/RConn2 -- GCB_1MVA/RConn2
  RELAY7/RConn3 -- GCB_1MVA/RConn3
  GCB_1MVA/LConn1 -- GenSet_1MVA_09082015/RConn1
  GCB_1MVA/LConn2 -- GenSet_1MVA_09082015/RConn2
  GCB_1MVA/LConn3 -- GenSet_1MVA_09082015/RConn3
  temp_2/LConn1 -- RELAY18/RConn1
  temp_2/LConn2 -- RELAY18/RConn2
  temp_2/LConn3 -- RELAY18/RConn3
  500kcmil_L15/LConn3 -- RELAY11/LConn3 -- 500kcmil_L002/RConn3
  500kcmil_L15/LConn2 -- RELAY11/LConn2 -- 500kcmil_L002/RConn2
  500kcmil_L15/LConn1 -- RELAY11/LConn1 -- 500kcmil_L002/RConn1
  RELAY12/RConn3 -- 500kcmil_L018/LConn3
  500kcmil_L15/RConn3 -- RELAY12/LConn3
  1/0AWG_cable1/LConn1 -- 2000 kVA3/RConn1
  RELAY11/RConn1 -- 1/0AWG_L022/LConn1
  RELAY11/RConn3 -- 1/0AWG_L022/LConn3
  500kcmil_L15/RConn1 -- RELAY12/LConn1
  RELAY12/RConn1 -- 500kcmil_L018/LConn1
  2000 kVA3/LConn1 -- 1/0AWG_L022/RConn1
  1/0AWG_cable1/RConn2 -- B004/LConn2
  RELAY3/LConn3 -- 500kcmil_L18/RConn3
  RELAY3/LConn1 -- 500kcmil_L18/RConn1
  RELAY3/LConn2 -- 500kcmil_L18/RConn2
  1/0AWG_cable1/RConn1 -- B004/LConn1
  2000 kVA3/LConn3 -- 1/0AWG_L022/RConn3
  RELAY12/LConn2 -- 500kcmil_L15/RConn2
  1/0AWG_cable1/LConn2 -- 2000 kVA3/RConn2
  1/0AWG_cable1/LConn3 -- 2000 kVA3/RConn3
  RELAY12/RConn2 -- 500kcmil_L018/LConn2
  RELAY11/RConn2 -- 1/0AWG_L022/LConn2
  1/0AWG_L022/RConn2 -- 2000 kVA3/LConn2
  1/0AWG_cable1/RConn3 -- B004/LConn3
  RELAY3/RConn3 -- 500kcmil_L002/LConn3
  RELAY3/RConn1 -- 500kcmil_L002/LConn1
  RELAY3/RConn2 -- 500kcmil_L002/LConn2
  500kcmil_L13/LConn1 -- 3750 kVA/RConn1
  3750 kVA/RConn2 -- 500kcmil_L13/LConn2
  500kcmil_L018/RConn2 -- 3750 kVA/LConn2
  500kcmil_L018/RConn1 -- 3750 kVA/LConn1
  500kcmil_L13/LConn3 -- 3750 kVA/RConn3
  500kcmil_L018/RConn3 -- 3750 kVA/LConn3
  4000 kVA/LConn1 -- Battery/RConn1
  4000 kVA/LConn2 -- Battery/RConn2
  4000 kVA/LConn3 -- Battery/RConn3

== system Model_DesktopSim/Battery ==
  1 - Enable 0 - Disable1 : Constant  Value=200
  1 - Enable 0 - Disable2 : Constant  Value=500
  1 - Enable 0 - Disable3 : Constant  Value=0
  Bus Selector : BusSelector  OutputSignals=Capacity,Bat Voltage
  HIL_BATT : Batt_lib/HIL_BATT
      link override Batt/Grid Tied Inverter/PLL_disc/PID Controller: SampleTime=Ts
  Scope : Scope
  Scope1 : Scope
  Scope2 : Scope
  A : PMIOPort  Port=1  Side=Right
  B : PMIOPort  Port=2  Side=Right
  C : PMIOPort  Port=3  Side=Right
  wires:
  1 - Enable 0 - Disable2/1 -> HIL_BATT/2
  HIL_BATT/1 -> Bus Selector/1  "Capacity"
  1 - Enable 0 - Disable1/1 -> HIL_BATT/1
  1 - Enable 0 - Disable3/1 -> HIL_BATT/3
  HIL_BATT/2 -> Scope1/1  "faults"
  Bus Selector/1 -> Scope/1  "<Capacity>"
  Bus Selector/2 -> Scope2/1  "<Bat Voltage>"
  connections:
  A/RConn1 -- HIL_BATT/RConn1
  B/RConn1 -- HIL_BATT/RConn2
  C/RConn1 -- HIL_BATT/RConn3

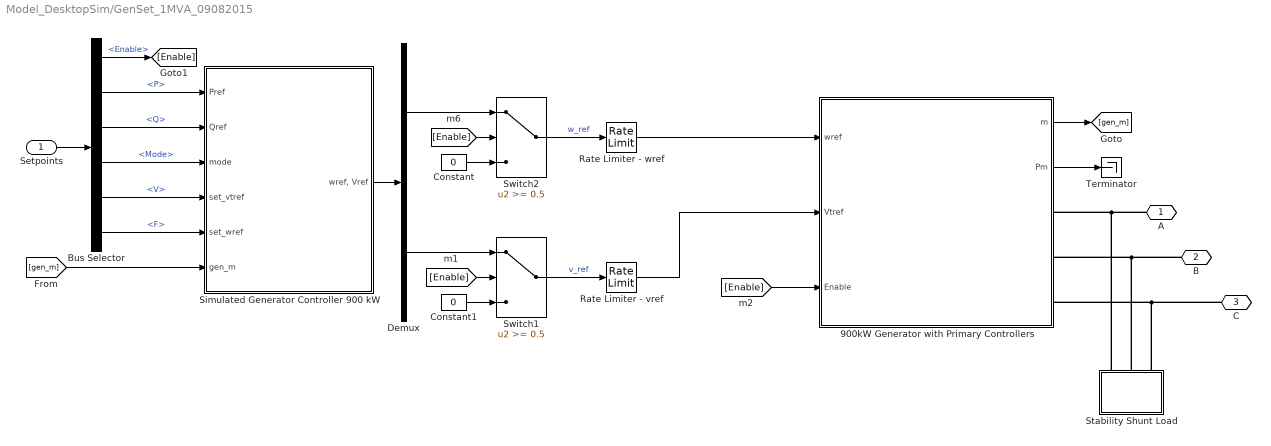
== system Model_DesktopSim/GenSet_1MVA_09082015 ==
  Setpoints : Inport
  900kW Generator with Primary Controllers : Subsystem
  Bus Selector : BusSelector  OutputSignals=Enable,P,Q,Mode,V,F
  Constant : Constant  Value=0
  Constant1 : Constant  Value=0
  Demux : Demux  Outputs=2
  Rate Limiter - vref : RateLimiter  RisingSlewLimit=0.5  FallingSlewLimit=-0.5  SampleTimeMode=inherited
  Rate Limiter - wref : RateLimiter  RisingSlewLimit=0.5  FallingSlewLimit=-0.5  SampleTimeMode=inherited
  Simulated Generator Controller 900 kW : Subsystem
  Stability Shunt Load : Subsystem  mask{v=460, kVA=80, pf=1}
  Switch1 : Switch  Threshold=0.5
  Switch2 : Switch  Threshold=0.5
  Terminator : Terminator
  A : PMIOPort  Port=1  Side=Right
  B : PMIOPort  Port=2  Side=Right
  C : PMIOPort  Port=3  Side=Right
  wires:
  Simulated Generator Controller 900 kW/1("wref, Vref") -> Demux/1
  Switch2/1 -> Rate Limiter - wref/1  "w_ref"
  Switch1/1 -> Rate Limiter - vref/1  "v_ref"
  Demux/1 -> Switch2/1
  Constant/1 -> Switch2/3
  Demux/2 -> Switch1/1
  Constant1/1 -> Switch1/3
  Rate Limiter - wref/1 -> 900kW Generator with Primary Controllers/1(wref)
  Rate Limiter - vref/1 -> 900kW Generator with Primary Controllers/2(Vtref)
  [Enable] -> Switch2/2
  [Enable] -> Switch1/2
  [Enable] -> 900kW Generator with Primary Controllers/3(Enable)
  900kW Generator with Primary Controllers/1(m) -> [gen_m]
  [gen_m] -> Simulated Generator Controller 900 kW/6(gen_m)
  900kW Generator with Primary Controllers/2(Pm) -> Terminator/1
  Setpoints/1 -> Bus Selector/1
  Bus Selector/6 -> Simulated Generator Controller 900 kW/5(set_wref)  "<F>"
  Bus Selector/5 -> Simulated Generator Controller 900 kW/4(set_vtref)  "<V>"
  Bus Selector/4 -> Simulated Generator Controller 900 kW/3(mode)  "<Mode>"
  Bus Selector/3 -> Simulated Generator Controller 900 kW/2(Qref)  "<Q>"
  Bus Selector/2 -> Simulated Generator Controller 900 kW/1(Pref)  "<P>"
  Bus Selector/1 -> [Enable]  "<Enable>"
  connections:
  A/RConn1 -- Stability Shunt Load/LConn1 -- 900kW Generator with Primary Controllers/RConn1
  B/RConn1 -- Stability Shunt Load/LConn2 -- 900kW Generator with Primary Controllers/RConn2
  C/RConn1 -- Stability Shunt Load/LConn3 -- 900kW Generator with Primary Controllers/RConn3

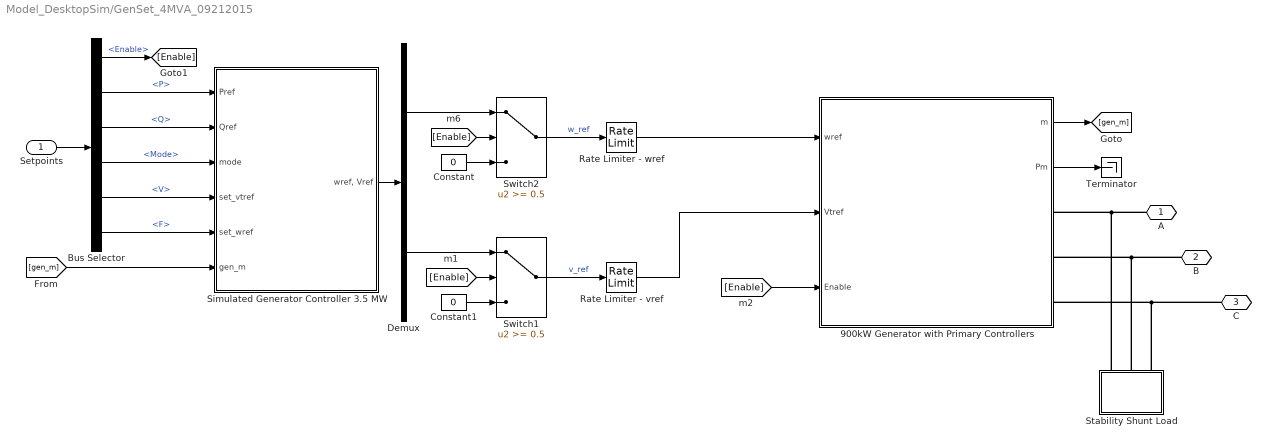
== system Model_DesktopSim/GenSet_4MVA_09212015 ==
  Setpoints : Inport
  900kW Generator with Primary Controllers : Subsystem
  Bus Selector : BusSelector  OutputSignals=Enable,P,Q,Mode,V,F
  Constant : Constant  Value=0
  Constant1 : Constant  Value=0
  Demux : Demux  Outputs=2
  Rate Limiter - vref : RateLimiter  RisingSlewLimit=0.5  FallingSlewLimit=-0.5  SampleTimeMode=inherited
  Rate Limiter - wref : RateLimiter  RisingSlewLimit=0.5  FallingSlewLimit=-0.5  SampleTimeMode=inherited
  Simulated Generator Controller 3.5 MW : Subsystem
  Stability Shunt Load : Subsystem  mask{v=460, kVA=80, pf=1}
  Switch1 : Switch  Threshold=0.5
  Switch2 : Switch  Threshold=0.5
  Terminator : Terminator
  A : PMIOPort  Port=1  Side=Right
  B : PMIOPort  Port=2  Side=Right
  C : PMIOPort  Port=3  Side=Right
  wires:
  Bus Selector/1 -> [Enable]  "<Enable>"
  Bus Selector/2 -> Simulated Generator Controller 3.5 MW/1(Pref)  "<P>"
  Bus Selector/3 -> Simulated Generator Controller 3.5 MW/2(Qref)  "<Q>"
  Bus Selector/4 -> Simulated Generator Controller 3.5 MW/3(mode)  "<Mode>"
  Bus Selector/5 -> Simulated Generator Controller 3.5 MW/4(set_vtref)  "<V>"
  Bus Selector/6 -> Simulated Generator Controller 3.5 MW/5(set_wref)  "<F>"
  Setpoints/1 -> Bus Selector/1
  900kW Generator with Primary Controllers/2(Pm) -> Terminator/1
  [gen_m] -> Simulated Generator Controller 3.5 MW/6(gen_m)
  900kW Generator with Primary Controllers/1(m) -> [gen_m]
  [Enable] -> 900kW Generator with Primary Controllers/3(Enable)
  [Enable] -> Switch1/2
  [Enable] -> Switch2/2
  Rate Limiter - vref/1 -> 900kW Generator with Primary Controllers/2(Vtref)
  Rate Limiter - wref/1 -> 900kW Generator with Primary Controllers/1(wref)
  Constant1/1 -> Switch1/3
  Demux/2 -> Switch1/1
  Constant/1 -> Switch2/3
  Demux/1 -> Switch2/1
  Switch1/1 -> Rate Limiter - vref/1  "v_ref"
  Switch2/1 -> Rate Limiter - wref/1  "w_ref"
  Simulated Generator Controller 3.5 MW/1("wref, Vref") -> Demux/1
  connections:
  Stability Shunt Load/LConn3 -- 900kW Generator with Primary Controllers/RConn3 -- C/RConn1
  Stability Shunt Load/LConn2 -- 900kW Generator with Primary Controllers/RConn2 -- B/RConn1
  Stability Shunt Load/LConn1 -- 900kW Generator with Primary Controllers/RConn1 -- A/RConn1

== system Model_DesktopSim/Gen_initial_condition_1MVA ==
  1 - PQ 2 - PV 3 - VF : Constant
  Bus Creator : BusCreator  Inputs=6
  DONOTCHANGE : Constant
  F : simulink/Math Operations/Slider Gain  low=0  gain=1  high=1
  P : simulink/Math Operations/Slider Gain  low=0  gain=0.8  high=1
  Q : simulink/Math Operations/Slider Gain  low=0  gain=0.2  high=0.5
  V : simulink/Math Operations/Slider Gain  low=0  gain=1  high=1
  e : Constant  Value=0
  S : Outport
  wires:
  1 - PQ 2 - PV 3 - VF/1 -> Bus Creator/5  "Mode"
  F/1 -> Bus Creator/4  "F"
  V/1 -> Bus Creator/3  "V"
  Q/1 -> Bus Creator/2  "Q"
  P/1 -> Bus Creator/1  "P"
  Bus Creator/1 -> S/1
  DONOTCHANGE/1 -> F/1, V/1, Q/1, P/1
  e/1 -> Bus Creator/6  "Enable"

== system Model_DesktopSim/Gen_initial_condition_4MVA ==
  1 - PQ 2 - PV 3 - VF : Constant
  Bus Creator : BusCreator  Inputs=6
  DONOTCHANGE : Constant
  F : simulink/Math Operations/Slider Gain  low=0  gain=1  high=1
  P : simulink/Math Operations/Slider Gain  low=0  gain=0.9  high=1
  Q : simulink/Math Operations/Slider Gain  low=0  gain=0.2  high=0.5
  V : simulink/Math Operations/Slider Gain  low=0  gain=1  high=1
  e : Constant  Value=0
  S : Outport
  wires:
  1 - PQ 2 - PV 3 - VF/1 -> Bus Creator/5  "Mode"
  F/1 -> Bus Creator/4  "F"
  V/1 -> Bus Creator/3  "V"
  Q/1 -> Bus Creator/2  "Q"
  P/1 -> Bus Creator/1  "P"
  Bus Creator/1 -> S/1
  DONOTCHANGE/1 -> F/1, V/1, Q/1, P/1
  e/1 -> Bus Creator/6  "Enable"

== system Model_DesktopSim/GenSet_1MVA_09082015/900kW Generator with Primary Controllers ==
  wref : Inport
  Vtref : Inport  Port=2
  Enable : Inport  Port=3
  Diesel Engine Speed & Voltage Control fast : Subsystem
  Synchronous Machine pu Fundamental : powerlib/Machines/Synchronous Machine pu Fundamental  PresetModel=22: 60Hz 460V 1075kVA 1800RPM  MechanicalLoad=Mechanical power Pm  ShowDetailedParameters=on  RotorType=Salient-pole  Units=per unit fundamental parameters  MeasurementBus=off  NominalParameters=[1.075e+06 460 60]  Stator=[0.01524 0.08 2.81 1.64]  Field=[0.004319 0.531]  Dampers2=[0.0652, 0.5134, 0.0287, 0.2553, 7.765e-3, 0.9167 ]  Dampers1=[0.2343 2.655 0.03365 0.2408]  Mechanical=[0.3222 0.01322 2]  PolePairs=2  InitialConditions="[ -99  0  0  0  0  0  0  0  0 ]"  SetSaturation=off  Saturation=[0.6404,0.7127,0.8441,0.9214,0.9956,1.082,1.19,1.316,1.457;0.7,0.7698,0.8872,0.9466,0.9969,1.046,1.1,1.151,1.201]  LoadFlowParameters=[1,0,0,0,0]  TsPowergui=0  TsBlock=-1  IterativeModel=Trapezoidal non iterative  IterativeDiscreteModel=Trapezoidal non iterative  BusType=swing  Pref=0  Qref=0  Qmin=-inf  Qmax=inf  PLF=0  QLF=0
  A : PMIOPort  Port=1  Side=Right
  B : PMIOPort  Port=2  Side=Right
  C : PMIOPort  Port=3  Side=Right
  m : Outport
  Pm : Outport  Port=2
  wires:
  Vtref/1 -> Diesel Engine Speed & Voltage Control fast/2(Vtref)
  wref/1 -> Diesel Engine Speed & Voltage Control fast/1(wref)
  Diesel Engine Speed & Voltage Control fast/2(Vf) -> Synchronous Machine pu Fundamental/2  "vf"
  Diesel Engine Speed & Voltage Control fast/1(Pm) -> Synchronous Machine pu Fundamental/1, Pm/1  "Pm"
  Enable/1 -> Diesel Engine Speed & Voltage Control fast/3(Generator Enable)
  Synchronous Machine pu Fundamental/1 -> Diesel Engine Speed & Voltage Control fast/4(m), m/1
  connections:
  C/RConn1 -- Synchronous Machine pu Fundamental/RConn3
  B/RConn1 -- Synchronous Machine pu Fundamental/RConn2
  A/RConn1 -- Synchronous Machine pu Fundamental/RConn1
